simulink model "ZZC_quadrotor_20230712 - 副本"  (R2019b)
settings: Solver=ode4  StartTime=0.0  StopTime=100  FixedStep=1e-4  RelTol=1e-3
libraries: simulink x1
settings Model: Creator=bitgar  LastModifiedBy=bitgar

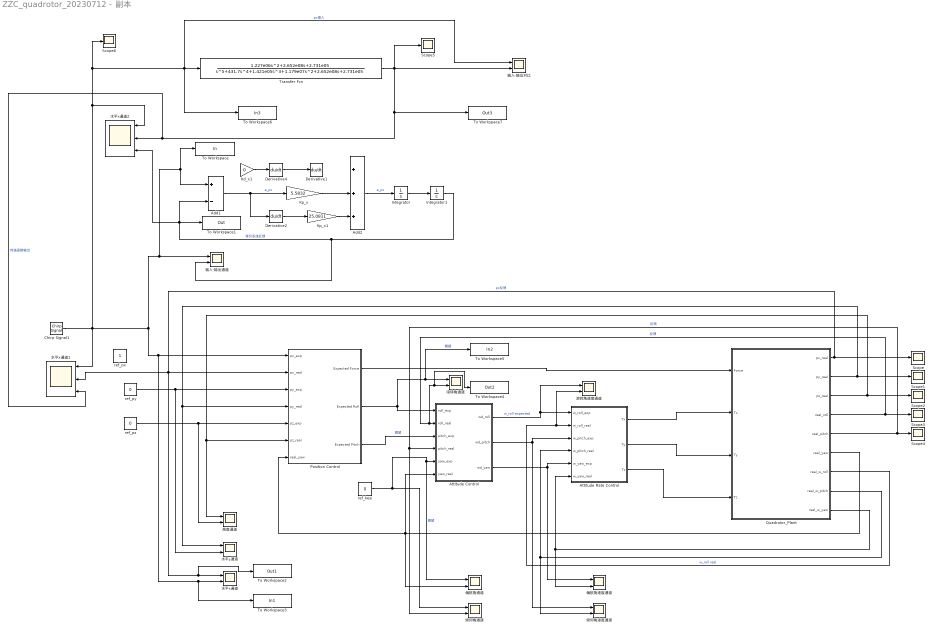
== system ZZC_quadrotor_20230712 - 副本 ==
  Add1 : Sum  Inputs=+-
  Add2 : Sum  Inputs=+++
  Attitude Control : Subsystem
  Attitude Rate Control : Subsystem
  Chirp Signal1 : simulink/Sources/Chirp Signal  f1=0.0001  T=100  f2=100
  Derivative1 : Derivative
  Derivative2 : Derivative
  Derivative4 : Derivative
  Integrator : Integrator
  Integrator1 : Integrator
  Kd_x1 : Gain  Gain=0
  Kp_x : Gain  Gain=5.5832
  Kp_x1 : Gain  Gain=25.0811
  Position Control : Subsystem
  Quadrotor_Plant : Subsystem
  Scope{,1..6} (7 alike) : Scope
  To Workspace : ToWorkspace  VariableName=In  SampleTime=-1
  To Workspace1 : ToWorkspace  VariableName=Out  SampleTime=-1
  To Workspace2 : ToWorkspace  VariableName=Out1  SampleTime=-1
  To Workspace3 : ToWorkspace  VariableName=In1  SampleTime=-1
  To Workspace4 : ToWorkspace  VariableName=Out2  SampleTime=-1
  To Workspace5 : ToWorkspace  VariableName=In2  SampleTime=-1
  To Workspace6 : ToWorkspace  VariableName=In3  SampleTime=-1
  To Workspace7 : ToWorkspace  VariableName=Out3  SampleTime=-1
  Transfer Fcn : TransferFcn  Numerator=[1.227e06 2.652e08 2.731e05]  Denominator=[1 431.7 1.421e05 1.179e07 2.652e08 2.731e05]
  ref_kesi : Constant  Value=0
  ref_px : Constant
  ref_py : Constant  Value=0
  ref_pz : Constant  Value=0
  俯仰角通道 : Scope  NumInputPorts=2
  俯仰角速度通道 : Scope  NumInputPorts=2
  偏航角通道 : Scope  NumInputPorts=2
  偏航角速度通道 : Scope  NumInputPorts=2
  水平x通道 : Scope  NumInputPorts=2
  水平x通道1 : Scope  NumInputPorts=3
  水平x通道2 : Scope  NumInputPorts=3
  水平y通道 : Scope  NumInputPorts=2
  滚转角通道 : Scope  NumInputPorts=2
  滚转角速度通道 : Scope  NumInputPorts=2
  输入-输出对比 : Scope  NumInputPorts=2
  输入-输出通道 : Scope  NumInputPorts=2
  高度通道 : Scope  NumInputPorts=2
  wires:
  Quadrotor_Plant/3(pz_real) -> 高度通道/1, Position Control/6(pz_real), Scope2/1
  Quadrotor_Plant/4(real_roll) -> Scope3/1, To Workspace4/1, 滚转角通道/2, Attitude Control/2(roll_real)  "反馈"
  Quadrotor_Plant/5(real_pitch) -> Scope4/1, 俯仰角通道/2, Attitude Control/4(pitch_real)  "反馈"
  Quadrotor_Plant/6(real_yaw) -> 偏航角通道/2, Position Control/7(real_yaw), Attitude Control/6(yaw_real)
  Attitude Control/2(wd_pitch) -> Attitude Rate Control/3(w_pitch_exp), 俯仰角速度通道/1
  Attitude Control/1(wd_roll) -> 滚转角速度通道/1, Attitude Rate Control/1(w_roll_exp)  "w_roll expected"
  ref_py/1 -> 水平y通道/2, Position Control/3(py_exp)
  Position Control/1(Expected Force) -> Quadrotor_Plant/1(Force)
  ref_pz/1 -> 高度通道/2, Position Control/5(pz_exp)
  ref_kesi/1 -> 俯仰角通道/1, 偏航角通道/1, Attitude Control/5(yaw_exp)  "期望"
  Quadrotor_Plant/2(py_real) -> 水平y通道/1, Position Control/4(py_real), Scope1/1
  Quadrotor_Plant/1(px_real) -> 水平x通道1/2, Position Control/2(px_real), To Workspace2/1, 水平x通道/1, Scope/1  "px反馈"
  Attitude Rate Control/1(Tx) -> Quadrotor_Plant/2(Tx)
  Attitude Rate Control/2(Ty) -> Quadrotor_Plant/3(Ty)
  Attitude Rate Control/3(Tz) -> Quadrotor_Plant/4(Tz)
  Quadrotor_Plant/7(real_w_roll) -> 滚转角速度通道/2, Attitude Rate Control/2(w_roll_real)  "w_roll real"
  Quadrotor_Plant/8(real_w_pitch) -> 俯仰角速度通道/2, Attitude Rate Control/4(w_pitch_real)
  Quadrotor_Plant/9(real_w_yaw) -> 偏航角速度通道/2, Attitude Rate Control/6(w_yaw_real)
  Attitude Control/3(wd_yaw) -> Attitude Rate Control/5(w_yaw_exp), 偏航角速度通道/1
  Kp_x/1 -> Add2/2
  Derivative4/1 -> Derivative1/1
  Derivative2/1 -> Kp_x1/1
  Kp_x1/1 -> Add2/3
  Add1/1 -> Derivative2/1, Kp_x/1  "e_px"
  Add2/1 -> Integrator/1  "e_px"
  Integrator/1 -> Integrator1/1
  Integrator1/1 -> 输入-输出通道/2, To Workspace1/1, 水平x通道2/3, Add1/2  "等价系统反馈"
  Kd_x1/1 -> Derivative4/1
  Chirp Signal1/1 -> Transfer Fcn/1, To Workspace6/1, 输入-输出对比/1, Scope6/1, 水平x通道2/1, 水平x通道1/1, Position Control/1(px_exp), To Workspace3/1, 水平x通道/2, To Workspace/1, Add1/1, 输入-输出通道/1  "px输入"
  Position Control/2(Expected Roll) -> To Workspace5/1, 滚转角通道/1, Attitude Control/1(roll_exp)  "期望"
  Position Control/3(Expected Pitch) -> Attitude Control/3(pitch_exp)  "期望"
  Transfer Fcn/1 -> 输入-输出对比/2, 水平x通道1/3, 水平x通道2/2, To Workspace7/1, Scope5/1  "传递函数输出"

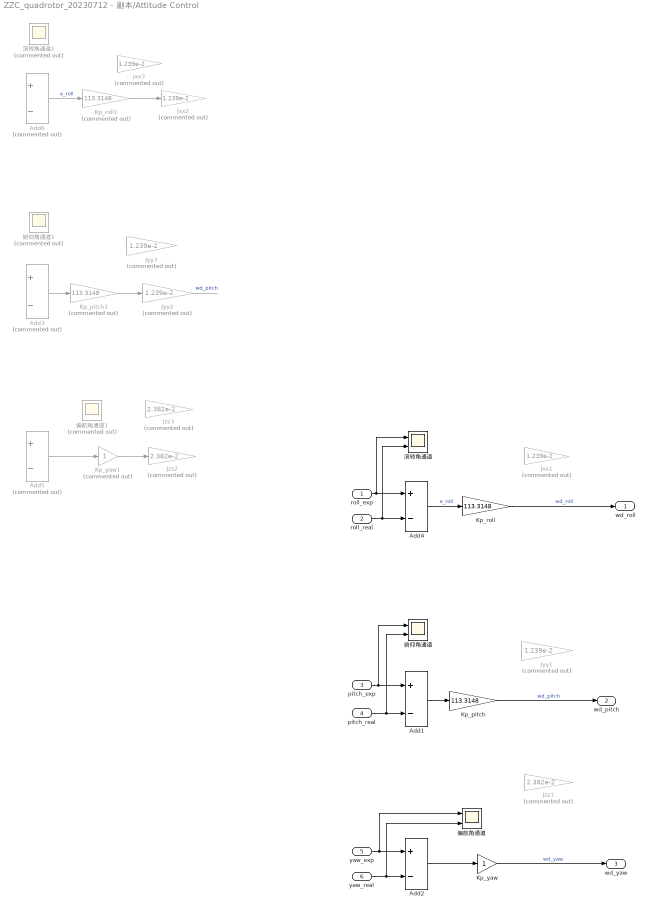
== system ZZC_quadrotor_20230712 - 副本/Attitude Control ==
  roll_exp : Inport
  roll_real : Inport  Port=2
  pitch_exp : Inport  Port=3
  pitch_real : Inport  Port=4
  yaw_exp : Inport  Port=5
  yaw_real : Inport  Port=6
  Add1 : Sum  Inputs=+-
  Add2 : Sum  Inputs=+-
  Add3 : Sum  Commented=on  Inputs=+-
  Add4 : Sum  Inputs=+-
  Add5 : Sum  Commented=on  Inputs=+-
  Add6 : Sum  Commented=on  Inputs=+-
  Jxx1 : Gain  Commented=on  Gain=1.239e-2
  Jxx2 : Gain  Commented=on  Gain=1.239e-2
  Jxx3 : Gain  Commented=on  Gain=1.239e-2
  Jyy1 : Gain  Commented=on  Gain=1.239e-2
  Jyy2 : Gain  Commented=on  Gain=1.239e-2
  Jyy3 : Gain  Commented=on  Gain=1.239e-2
  Jzz1 : Gain  Commented=on  Gain=2.382e-2
  Jzz2 : Gain  Commented=on  Gain=2.382e-2
  Jzz3 : Gain  Commented=on  Gain=2.382e-2
  Kp_pitch : Gain  Gain=113.3148
  Kp_pitch1 : Gain  Commented=on  Gain=113.3148
  Kp_roll : Gain  Gain=113.3148
  Kp_roll1 : Gain  Commented=on  Gain=113.3148
  Kp_yaw : Gain
  Kp_yaw1 : Gain  Commented=on
  俯仰角通道 : Scope  NumInputPorts=2
  俯仰角通道1 : Scope  Commented=on  NumInputPorts=2
  偏航角通道 : Scope  NumInputPorts=2
  偏航角通道1 : Scope  Commented=on  NumInputPorts=2
  滚转角通道 : Scope  NumInputPorts=2
  滚转角通道1 : Scope  Commented=on  NumInputPorts=2
  wd_roll : Outport
  wd_pitch : Outport  Port=2
  wd_yaw : Outport  Port=3
  wires:
  roll_exp/1 -> 滚转角通道/1, Add4/1
  roll_real/1 -> 滚转角通道/2, Add4/2
  pitch_exp/1 -> 俯仰角通道/1, Add1/1
  pitch_real/1 -> 俯仰角通道/2, Add1/2
  yaw_real/1 -> 偏航角通道/2, Add2/2
  Add4/1 -> Kp_roll/1  "e_roll"
  yaw_exp/1 -> 偏航角通道/1, Add2/1
  Add1/1 -> Kp_pitch/1
  Add2/1 -> Kp_yaw/1
  Kp_roll/1 -> wd_roll/1  "wd_roll"
  Kp_pitch/1 -> wd_pitch/1  "wd_pitch"
  Kp_yaw/1 -> wd_yaw/1  "wd_yaw"
  Kp_yaw1/1 -> Jzz2/1
  Add3/1 -> Kp_pitch1/1
  Add6/1 -> Kp_roll1/1  "e_roll"
  Kp_roll1/1 -> Jxx2/1
  Kp_pitch1/1 -> Jyy2/1
  Jyy2/1 -> ?  "wd_pitch"
  Add5/1 -> Kp_yaw1/1

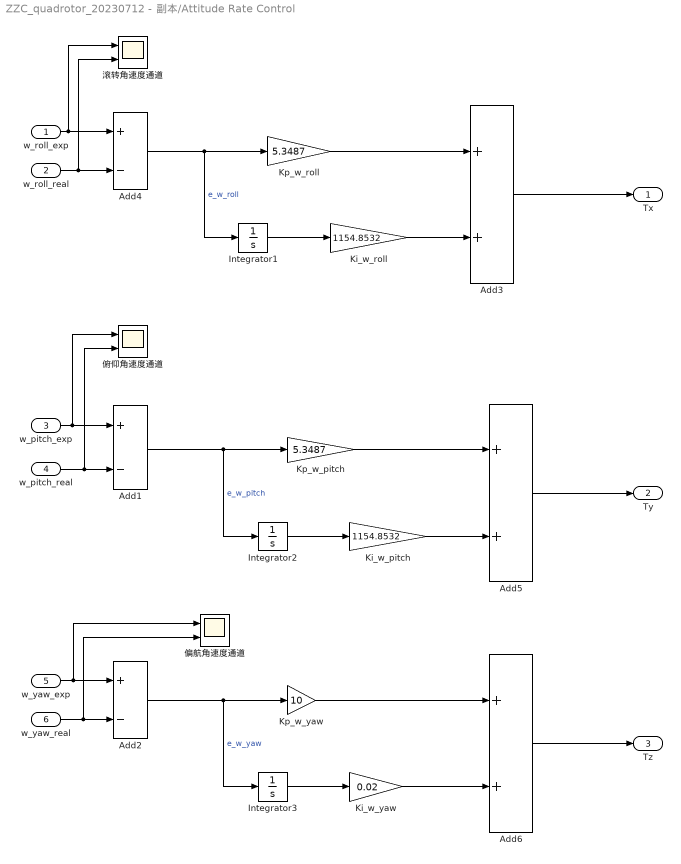
== system ZZC_quadrotor_20230712 - 副本/Attitude Rate Control ==
  w_roll_exp : Inport
  w_roll_real : Inport  Port=2
  w_pitch_exp : Inport  Port=3
  w_pitch_real : Inport  Port=4
  w_yaw_exp : Inport  Port=5
  w_yaw_real : Inport  Port=6
  Add1 : Sum  Inputs=+-
  Add2 : Sum  Inputs=+-
  Add3 : Sum
  Add4 : Sum  Inputs=+-
  Add5 : Sum
  Add6 : Sum
  Integrator1 : Integrator
  Integrator2 : Integrator
  Integrator3 : Integrator
  Ki_w_pitch : Gain  Gain=1154.8532
  Ki_w_roll : Gain  Gain=1154.8532
  Ki_w_yaw : Gain  Gain=0.02
  Kp_w_pitch : Gain  Gain=5.3487
  Kp_w_roll : Gain  Gain=5.3487
  Kp_w_yaw : Gain  Gain=10
  俯仰角速度通道 : Scope  NumInputPorts=2
  偏航角速度通道 : Scope  NumInputPorts=2
  滚转角速度通道 : Scope  NumInputPorts=2
  Tx : Outport
  Ty : Outport  Port=2
  Tz : Outport  Port=3
  wires:
  w_roll_exp/1 -> 滚转角速度通道/1, Add4/1
  w_roll_real/1 -> 滚转角速度通道/2, Add4/2
  w_pitch_exp/1 -> 俯仰角速度通道/1, Add1/1
  w_pitch_real/1 -> 俯仰角速度通道/2, Add1/2
  w_yaw_real/1 -> 偏航角速度通道/2, Add2/2
  Add4/1 -> Integrator1/1, Kp_w_roll/1  "e_w_roll"
  w_yaw_exp/1 -> 偏航角速度通道/1, Add2/1
  Add3/1 -> Tx/1
  Ki_w_roll/1 -> Add3/2
  Kp_w_roll/1 -> Add3/1
  Integrator1/1 -> Ki_w_roll/1
  Integrator2/1 -> Ki_w_pitch/1
  Kp_w_pitch/1 -> Add5/1
  Ki_w_pitch/1 -> Add5/2
  Add1/1 -> Integrator2/1, Kp_w_pitch/1  "e_w_pitch"
  Add5/1 -> Ty/1
  Add2/1 -> Integrator3/1, Kp_w_yaw/1  "e_w_yaw"
  Integrator3/1 -> Ki_w_yaw/1
  Kp_w_yaw/1 -> Add6/1
  Ki_w_yaw/1 -> Add6/2
  Add6/1 -> Tz/1

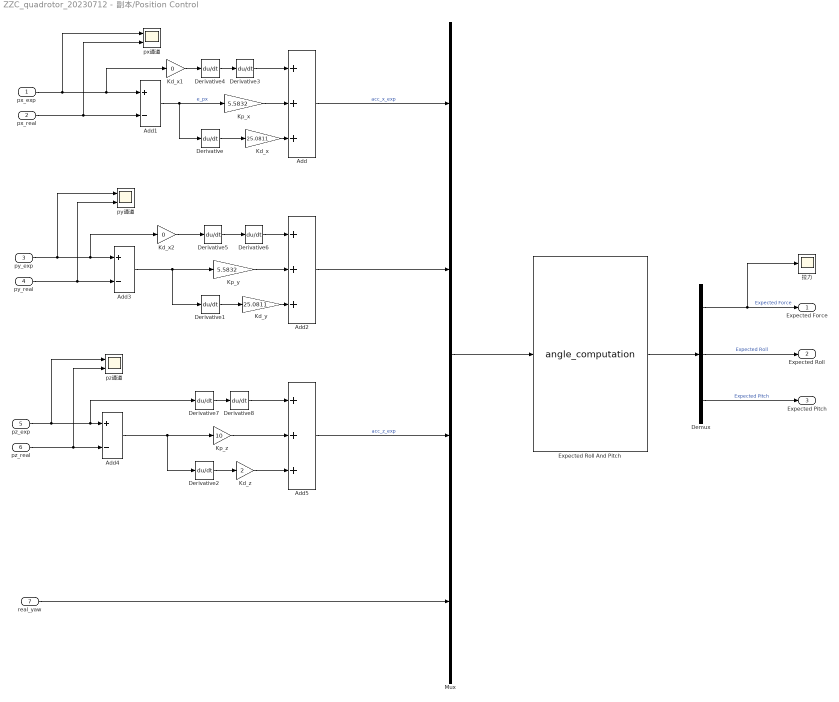
== system ZZC_quadrotor_20230712 - 副本/Position Control ==
  px_exp : Inport
  px_real : Inport  Port=2
  py_exp : Inport  Port=3
  py_real : Inport  Port=4
  pz_exp : Inport  Port=5
  pz_real : Inport  Port=6
  real_yaw : Inport  Port=7
  Add : Sum  Inputs=3
  Add1 : Sum  Inputs=+-
  Add2 : Sum  Inputs=3
  Add3 : Sum  Inputs=+-
  Add4 : Sum  Inputs=+-
  Add5 : Sum  Inputs=3
  Demux : Demux  Outputs=3
  Derivative{,1..8} (9 alike) : Derivative
  Expected Roll And Pitch : S-Function  FunctionName=angle_computation  Parameters=1 9.81  SFunctionDeploymentMode=off  EnableBusSupport=off
  Kd_x : Gain  Gain=25.0811
  Kd_x1 : Gain  Gain=0
  Kd_x2 : Gain  Gain=0
  Kd_y : Gain  Gain=25.0811
  Kd_z : Gain  Gain=2
  Kp_x : Gain  Gain=5.5832
  Kp_y : Gain  Gain=5.5832
  Kp_z : Gain  Gain=10
  Mux : Mux
  px通道 : Scope  NumInputPorts=2
  py通道 : Scope  NumInputPorts=2
  pz通道 : Scope  NumInputPorts=2
  拉力 : Scope
  Expected Force : Outport
  Expected Roll : Outport  Port=2
  Expected Pitch : Outport  Port=3
  wires:
  Add1/1 -> Derivative/1, Kp_x/1  "e_px"
  Mux/1 -> Expected Roll And Pitch/1
  Expected Roll And Pitch/1 -> Demux/1
  Demux/2 -> Expected Roll/1  "Expected Roll"
  Demux/3 -> Expected Pitch/1  "Expected Pitch"
  px_exp/1 -> Kd_x1/1, Add1/1, px通道/1
  Derivative/1 -> Kd_x/1
  Kd_x/1 -> Add/3
  px_real/1 -> Add1/2, px通道/2
  Kp_x/1 -> Add/2
  Kd_y/1 -> Add2/3
  Add3/1 -> Derivative1/1, Kp_y/1
  Derivative1/1 -> Kd_y/1
  Kd_z/1 -> Add5/3
  Add4/1 -> Derivative2/1, Kp_z/1
  Derivative2/1 -> Kd_z/1
  py_exp/1 -> Kd_x2/1, Add3/1, py通道/1
  py_real/1 -> Add3/2, py通道/2
  pz_exp/1 -> pz通道/1, Derivative7/1, Add4/1
  pz_real/1 -> Add4/2, pz通道/2
  Demux/1 -> 拉力/1, Expected Force/1  "Expected Force"
  Add5/1 -> Mux/3  "acc_z_exp"
  Add2/1 -> Mux/2
  Add/1 -> Mux/1  "acc_x_exp"
  Derivative4/1 -> Derivative3/1
  Derivative3/1 -> Add/1
  Kp_y/1 -> Add2/2
  Derivative5/1 -> Derivative6/1
  Derivative6/1 -> Add2/1
  Kp_z/1 -> Add5/2
  Derivative7/1 -> Derivative8/1
  Derivative8/1 -> Add5/1
  real_yaw/1 -> Mux/4
  Kd_x1/1 -> Derivative4/1
  Kd_x2/1 -> Derivative5/1

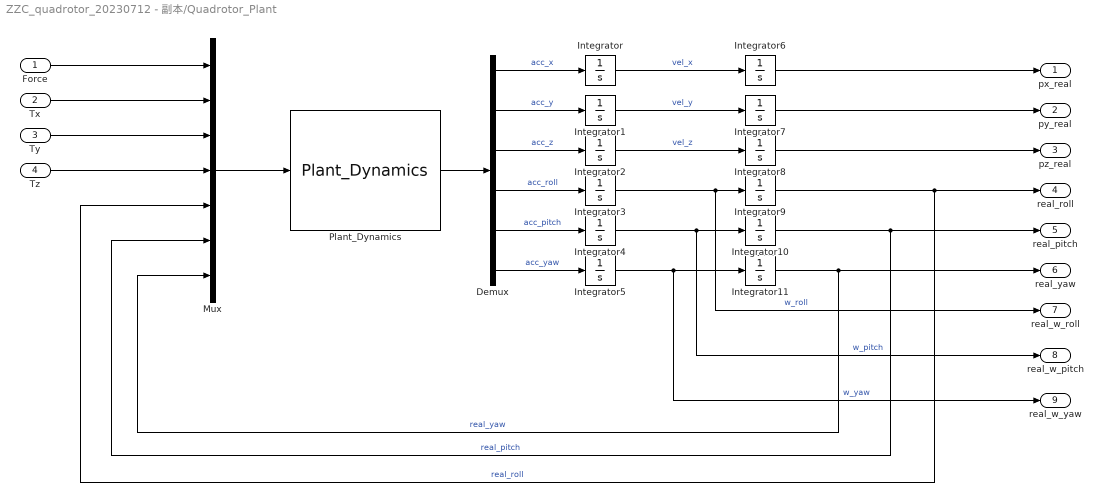
== system ZZC_quadrotor_20230712 - 副本/Quadrotor_Plant ==
  Force : Inport
  Tx : Inport  Port=2
  Ty : Inport  Port=3
  Tz : Inport  Port=4
  Demux : Demux  Outputs=6
  Integrator{,1..11} (12 alike) : Integrator
  Mux : Mux  Inputs=7
  Plant_Dynamics : S-Function  FunctionName=Plant_Dynamics  Parameters=1 9.81 0.01239 0.01239 0.02382  SFunctionDeploymentMode=off  EnableBusSupport=off
  px_real : Outport
  py_real : Outport  Port=2
  pz_real : Outport  Port=3
  real_roll : Outport  Port=4
  real_pitch : Outport  Port=5
  real_yaw : Outport  Port=6
  real_w_roll : Outport  Port=7
  real_w_pitch : Outport  Port=8
  real_w_yaw : Outport  Port=9
  wires:
  Demux/4 -> Integrator3/1  "acc_roll"
  Integrator6/1 -> px_real/1
  Mux/1 -> Plant_Dynamics/1
  Demux/3 -> Integrator2/1  "acc_z"
  Integrator/1 -> Integrator6/1  "vel_x"
  Tx/1 -> Mux/2
  Integrator1/1 -> Integrator7/1  "vel_y"
  Demux/1 -> Integrator/1  "acc_x"
  Integrator8/1 -> pz_real/1
  Demux/5 -> Integrator4/1  "acc_pitch"
  Demux/6 -> Integrator5/1  "acc_yaw"
  Integrator2/1 -> Integrator8/1  "vel_z"
  Demux/2 -> Integrator1/1  "acc_y"
  Tz/1 -> Mux/4
  Integrator7/1 -> py_real/1
  Force/1 -> Mux/1
  Ty/1 -> Mux/3
  Integrator9/1 -> real_roll/1, Mux/5  "real_roll"
  Integrator10/1 -> real_pitch/1, Mux/6  "real_pitch"
  Plant_Dynamics/1 -> Demux/1
  Integrator11/1 -> real_yaw/1, Mux/7  "real_yaw"
  Integrator3/1 -> real_w_roll/1, Integrator9/1  "w_roll"
  Integrator4/1 -> real_w_pitch/1, Integrator10/1  "w_pitch"
  Integrator5/1 -> real_w_yaw/1, Integrator11/1  "w_yaw"
